simulink model "RCAM_OP1_LONG"  (R2022b)
settings: Solver=VariableStepAuto  StartTime=0.0  StopTime=Tsim  RelTol=1e-3
values from neighbouring files (symbols this model uses):
  Elevator_doublet = 1    [Autopilot_Design_Script.m]
libraries: simulink_extras x1, cstblocks x1
settings Model: Creator=bendr  LastModifiedBy=bendr

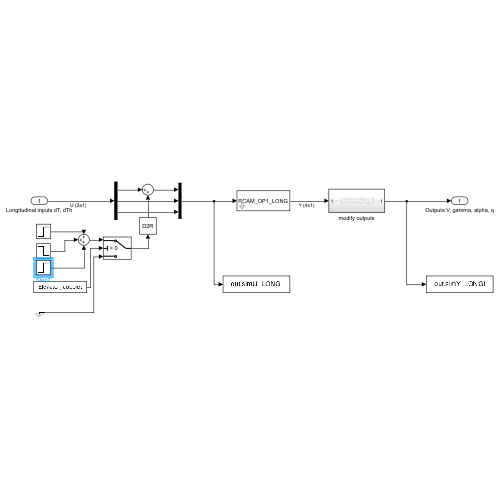
[thumbnail: Simulink's stored preview of the top-level diagram]
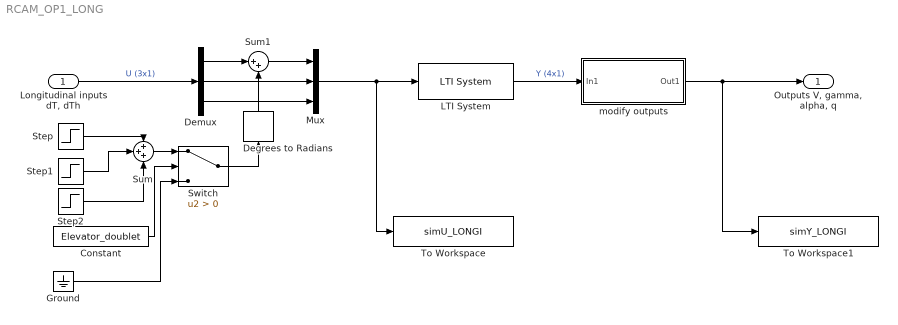
== system RCAM_OP1_LONG ==
  "Longitudinal inputs dT, dTh" : Inport
  Constant : Constant  Value=Elevator_doublet
  Degrees to Radians : simulink_extras/Transformations/Degrees to Radians
  Demux : Demux  Outputs=3
  Ground : Ground
  LTI System : cstblocks/LTI System  sys=RCAM_OP1_LONG  IC=[]
  Mux : Mux  Inputs=3
  Step : Step  SampleTime=0
  Step1 : Step  Time=6  After=-2  SampleTime=0
  Step2 : Step  Time=11  SampleTime=0
  Sum : Sum  Inputs=+++
  Sum1 : Sum  Inputs=|++
  Switch : Switch  Criteria=u2 > Threshold  SaturateOnIntegerOverflow=off  InputSameDT=off
  To Workspace : ToWorkspace  VariableName=simU_LONGI  SaveFormat=Timeseries  SampleTime=-1
  To Workspace1 : ToWorkspace  VariableName=simY_LONGI  SaveFormat=Timeseries  SampleTime=-1
  modify outputs : Subsystem
  "Outputs V, gamma, alpha, q" : Outport
  wires:
  LTI System/1 -> modify outputs/1(In1)  "Y (4x1)"
  modify outputs/1(Out1) -> "Outputs V, gamma, alpha, q"/1, To Workspace1/1
  Step/1 -> Sum/1
  Sum/1 -> Switch/1
  Step1/1 -> Sum/2
  "Longitudinal inputs dT, dTh"/1 -> Demux/1  "U (3x1)"
  Ground/1 -> Switch/3
  Demux/1 -> Sum1/1
  Switch/1 -> Degrees to Radians/1
  Constant/1 -> Switch/2
  Mux/1 -> To Workspace/1, LTI System/1
  Sum1/1 -> Mux/1
  Demux/2 -> Mux/2
  Demux/3 -> Mux/3
  Degrees to Radians/1 -> Sum1/2
  Step2/1 -> Sum/3

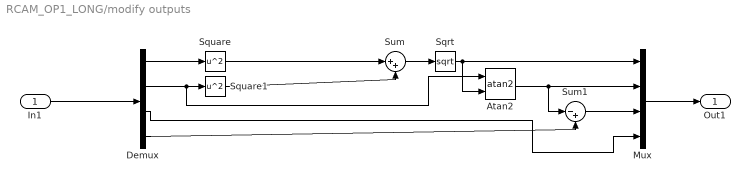
== system RCAM_OP1_LONG/modify outputs ==
  In1 : Inport
  Atan2 : Trigonometry  Operator=atan2
  Demux : Demux
  Mux : Mux
  Sqrt : Sqrt
  Square : Math  Operator=square
  Square1 : Math  Operator=square
  Sum : Sum  Inputs=|++
  Sum1 : Sum  Inputs=|-+
  Out1 : Outport
  wires:
  In1/1 -> Demux/1
  Mux/1 -> Out1/1
  Demux/1 -> Square/1
  Demux/2 -> Atan2/1, Square1/1
  Square/1 -> Sum/1
  Square1/1 -> Sum/2
  Sqrt/1 -> Atan2/2, Mux/1
  Sum/1 -> Sqrt/1
  Atan2/1 -> Sum1/1, Mux/2
  Sum1/1 -> Mux/3
  Demux/4 -> Sum1/2
  Demux/3 -> Mux/4
